simulink model "SDOF_LINER__model"  (R2021a)
settings: Solver=VariableStepAuto  StartTime=0.0  StopTime=1  RelTol=1e-3
values from neighbouring files (symbols this model uses):
  A_pinc = 1    [params.m]
  c0 = 344.5389    [XX_SDOF_LINER__TimeDomain.m]    (also in params.m)
  Ca = Vb/1/rho/c0^2/Sd1*1    [XX_SDOF_LINER__TimeDomain.m]    (also in params.m = (V/(rho0*c0^2))/S)
  Cac = Cmc*Sd    (= 2.0742e-07)    [XX_SDOF_LINER__TimeDomain.m]    (also in params.m = 2.04827190652e-07)
  f = linspace(0,1,NFFT/2+1)/2/dt    [XX_SDOF_LINER__TimeDomain.m]
  Ma = Vb/2*rho/Sd1*1    [XX_SDOF_LINER__TimeDomain.m]    (also in params.m = rho0*V/S)
  Mas = Mms/Sd    (= 0.494666666667)    [XX_SDOF_LINER__TimeDomain.m]    (also in params.m)
  Ras = Rms/Sd    (= 294.083333333)    [XX_SDOF_LINER__TimeDomain.m]    (also in params.m)
  rho0 = 1.1965    [params.m]
  S = amp*sin(2*pi*freq*time)    [SDOF_LINER__TimeDomain.m]    (also in params.m = h*sqrt(Sd))
  Sd = 12e-4    (= 0.0012)    [XX_SDOF_LINER__TimeDomain.m]    (also in params.m)
  ts = 1/fs    (= 2e-06)    [SDOF_LINER__TimeDomain.m]    (also in SDOF_LINER__TimeDomain_SL.m = 1e-05)
settings Model: Creator=padlewsk  LastModifiedBy=padlewsk

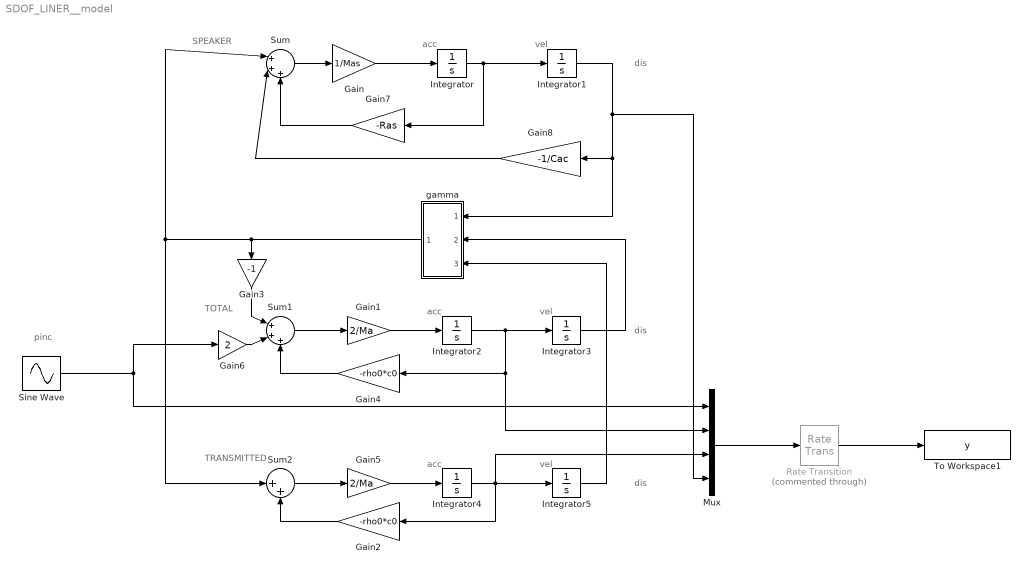
== system SDOF_LINER__model ==
  note: TRANSMITTED
  note: pinc
  note: acc
  note: vel
  note: dis
  note: vel
  note: acc
  note: vel
  note: acc
  note: SPEAKER
  note: TOTAL
  note: dis
  note: dis
  Gain : Gain  Gain=1/Mas
  Gain1 : Gain  Gain=2/Ma
  Gain2 : Gain  Gain=-rho0*c0
  Gain3 : Gain  Gain=-1
  Gain4 : Gain  Gain=-rho0*c0
  Gain5 : Gain  Gain=2/Ma
  Gain6 : Gain  Gain=2
  Gain7 : Gain  Gain=-Ras
  Gain8 : Gain  Gain=-1/Cac
  Integrator{,1..5} (6 alike) : Integrator
  Mux : Mux
  Rate Transition : RateTransition  Commented=through  OutPortSampleTime=ts
  Sine Wave : Sin  Amplitude=A_pinc  Frequency=2*pi*f  SampleTime=ts
  Sum : Sum  Inputs=|+++
  Sum1 : Sum  Inputs=|+++
  Sum2 : Sum  Inputs=|++
  To Workspace1 : ToWorkspace  VariableName=y  SaveFormat=Timeseries  SampleTime=ts
  gamma : Subsystem
  wires:
  Integrator/1 -> Gain7/1, Integrator1/1
  Sum/1 -> Gain/1
  Sum1/1 -> Gain1/1
  Integrator2/1 -> Mux/2, Gain4/1, Integrator3/1
  Sum2/1 -> Gain5/1
  Integrator4/1 -> Gain2/1, Mux/3, Integrator5/1
  Gain/1 -> Integrator/1
  Gain1/1 -> Integrator2/1
  Integrator1/1 -> Mux/4, Gain8/1, gamma/1(In1)
  Gain8/1 -> Sum/2
  gamma/1(Out1) -> Gain3/1, Sum2/1, Sum/1
  Gain3/1 -> Sum1/1
  Gain4/1 -> Sum1/3
  Gain5/1 -> Integrator4/1
  Gain2/1 -> Sum2/2
  Sine Wave/1 -> Mux/1, Gain6/1
  Gain6/1 -> Sum1/2
  Integrator5/1 -> gamma/3(In3)
  Integrator3/1 -> gamma/2(In2)
  Gain7/1 -> Sum/3
  Mux/1 -> Rate Transition/1
  Rate Transition/1 -> To Workspace1/1

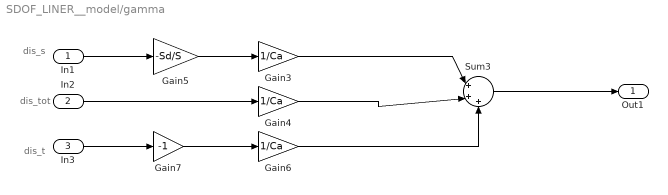
== system SDOF_LINER__model/gamma ==
  note: dis_s
  note: dis_tot
  note: dis_t
  In1 : Inport
  In2 : Inport  Port=2
  In3 : Inport  Port=3
  Gain3 : Gain  Gain=1/Ca
  Gain4 : Gain  Gain=1/Ca
  Gain5 : Gain  Gain=-Sd/S
  Gain6 : Gain  Gain=1/Ca
  Gain7 : Gain  Gain=-1
  Sum3 : Sum  Inputs=|+++
  Out1 : Outport
  wires:
  Gain6/1 -> Sum3/3
  Gain7/1 -> Gain6/1
  Gain4/1 -> Sum3/2
  Gain3/1 -> Sum3/1
  Sum3/1 -> Out1/1
  Gain5/1 -> Gain3/1
  In3/1 -> Gain7/1
  In2/1 -> Gain4/1
  In1/1 -> Gain5/1
